simulink model "SMC_STA_HW_2_r2024b_test_2024"  (R2024b)
settings: Solver=FixedStepDiscrete  StartTime=0.0  StopTime=inf  FixedStep=0.002  RelTol=1e-3  EnableMultiTasking=on
PostLoadFcn:
  | qc_set_target_type(getConfigSet(bdroot, 'QUARC Default Target Configuration'));
undefined symbols (not defined in the file): HIL
libraries: quarc_library x4
settings Model: SimulationMode=external  ExtModeTrigDuration=5000  Creator=pmartin  LastModifiedBy=U448565
settings SolverCC: AlgebraicLoopSolver=TrustRegion  PositivePriorityOrder=on
settings DataIOCC: LimitDataPoints=on  SaveFormat=Array  SignalLoggingSaveFormat=ModelDataLogs  ReturnWorkspaceOutputs=off
settings OptimizationCC: ExpressionDepthLimit=2147483647  InitFltsAndDblsToZero=on
settings DebuggingCC: SaveWithParameterizedLinksMsg=none  UnderspecifiedInitializationDetection=Classic  MergeDetectMultiDrivingBlocksExec=none  SolverPrmCheckMsg=warning  MultiTaskDSMMsg=warning  MultiTaskCondExecSysMsg=none  FcnCallInpInsideContextMsg=warning  UnconnectedInputMsg=warning  UnconnectedOutputMsg=warning  UnconnectedLineMsg=warning  StateNameClashWarn=warning  SFUnexpectedBacktrackingDiag=warning  SFNoUnconditionalDefaultTransitionDiag=warning  SFExecutionAtInitializationDiag=none  ArithmeticOperatorsInVariantConditions=warning
settings ModelReferenceCC: PropagateSignalLabelsOutOfModel=off
settings SFSimCC: SimUseLocalCustomCode=off  CustomCodeUndefinedFunction=UseInterfaceOnly
settings RTWCC: Description=QUARC Win64 Target Using Toolchain  SystemTargetFile=quarc_win64.tlc  TemplateMakefile=quarc_default_tmf  RTWUseLocalCustomCode=off  Toolchain=QUARC win64 | nmake (64-bit Windows)  BuildConfiguration=Faster Runs  GPUComputeCapability=3.5
settings CodeAppCC: StateflowObjectComments=on
settings STFCustomTargetCC: ConcurrentExecutionCompliant=on  GRTInterface=on  UseToolchainInfoCompliant=on  SystemTargetFile=quarc_win64.tlc
settings GRTTargetCC: TargetLangStandard=C89/C90 (ANSI)  ParMdlRefBuildCompliant=off  CompOptLevelCompliant=off  CombineOutputUpdateFcns=off  MatFileLogging=off  CPPClassGenCompliant=off  GRTInterface=on  ExtMode=on  ExtModeMexFile=quarc_comm
settings ConfigComp: CovMetricSettings=dw  CovSaveCumulativeToWorkspaceVar=on  CovSaveSingleToWorkspaceVar=on  CovExternalEMLEnable=off  CovBoundaryAbsTol=1.0e-5

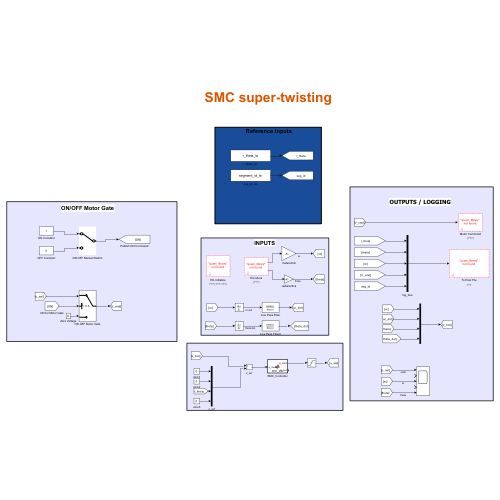
[thumbnail: Simulink's stored preview of the top-level diagram]
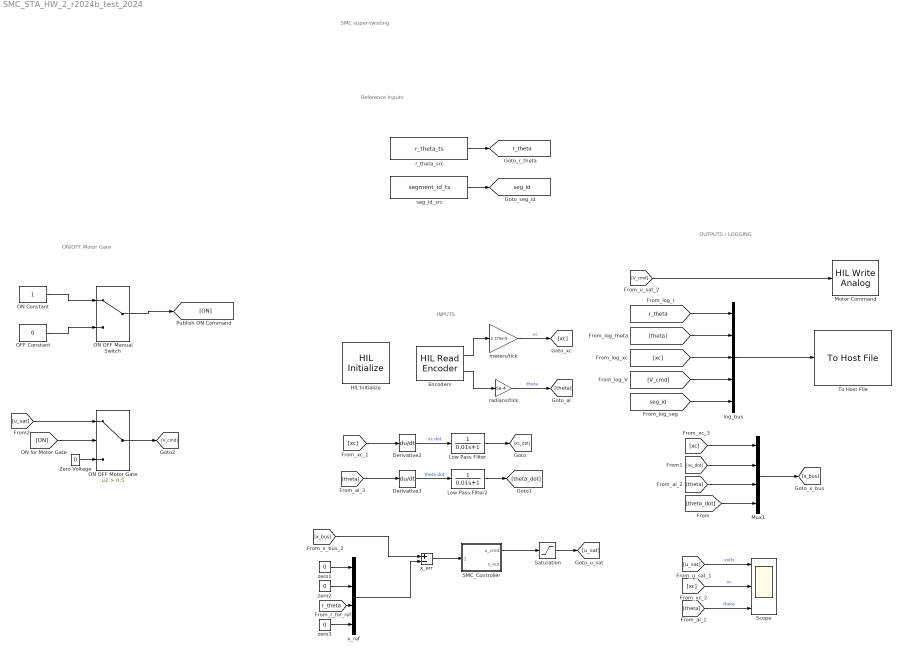
== system SMC_STA_HW_2_r2024b_test_2024 ==
  note: OUTPUTS / LOGGING
  note: INPUTS
  note: SMC super-twisting
  note: Reference Inputs
  note: ON/OFF Motor Gate
  Derivative2 : Derivative
  Derivative3 : Derivative
  Encoders : quarc_library/Data Acquisition/Generic/Immediate I//O/HIL Read Encoder  object_name=HIL-1  channels=[0:1]  sample_time=qc_get_step_size  active=on  vector_output=off  data_type_mode=Inherit via back propagation  data_type=double
  HIL Initialize : quarc_library/Data Acquisition/Generic/Configuration/HIL Initialize  object_name=HIL-1  board_type=q2_usb  board_number=0  board_options=d0=digital;d1=digital;led=auto;update_rate=normal  exclusive=off  active=off  hardware_clocks=[0:2]  clock_modes=[]  initial_clock_frequencies=[]  set_clock_params_at_start=off  set_clock_params_at_switch_in=off  set_clock_frequencies_at_start=off  set_clock_frequencies_at_switch_in=off  analog_input_channels=[0:1]  analog_input_configurations=[]  analog_input_maximums=10  analog_input_minimums=-10  set_analog_input_params_at_start=on  set_analog_input_params_at_switch_in=off  analog_output_channels=[0:1]  analog_output_maximums=10  analog_output_minimums=-10  initial_analog_outputs=[0]  final_analog_outputs=[0]  watchdog_analog_outputs=0  set_analog_output_params_at_start=on  set_analog_output_params_at_switch_in=off  set_analog_outputs_at_start=on  set_analog_outputs_at_switch_in=off  set_analog_outputs_at_terminate=on  set_analog_outputs_at_switch_out=off  set_analog_outputs_on_watchdog=off  digital_input_channels=[]  digital_output_channels=[0:7]  digital_output_configuration=[]  initial_digital_outputs=[0]  final_digital_outputs=[0]  watchdog_digital_outputs=[0]  set_digital_output_params_at_start=off  set_digital_output_params_at_switch_in=off  set_digital_outputs_at_start=on  set_digital_outputs_at_switch_in=off  set_digital_outputs_at_terminate=on  set_digital_outputs_at_switch_out=off  set_digital_outputs_on_watchdog=off  encoder_channels=[0:1]  quadrature=[4]  encoder_filter_frequency=[]  initial_encoder_counts=[0]  set_encoder_params_at_start=on  set_encoder_params_at_switch_in=off  set_encoder_counts_at_start=on  set_encoder_counts_at_switch_in=off  pwm_channels=[]  pwm_modes=[0]  pwm_frequency=1/0.020  pwm_configuration=[]  pwm_alignment=[]  pwm_polarity=[]  pwm_leading_deadband=[]  pwm_trailing_deadband=[]  initial_pwm_outputs=[0]  final_pwm_outputs=[0]  watchdog_pwm_outputs=[0]  set_pwm_params_at_start=on  set_pwm_params_at_switch_in=off  set_pwm_outputs_at_start=on  set_pwm_outputs_at_switch_in=off  set_pwm_outputs_at_terminate=on  set_pwm_outputs_at_switch_out=off  set_pwm_outputs_on_watchdog=off  other_output_channels=[]  initial_other_outputs=[]  final_other_outputs=[]  watchdog_other_outputs=[]  set_other_outputs_at_start=off  set_other_outputs_at_switch_in=off  set_other_outputs_at_terminate=off  set_other_outputs_at_switch_out=off  set_other_outputs_on_watchdog=off
  Low Pass Filter : TransferFcn  Denominator=[0.01 1]
  Low Pass Filter2 : TransferFcn  Denominator=[0.01 1]
  Motor Command : quarc_library/Data Acquisition/Generic/Immediate I//O/HIL Write Analog  object_name=HIL-1  channels=0  sample_time=-1  active=off  vector_input=off
  Mux1 : Mux
  OFF Constant : Constant  Value=0
  ON Constant : Constant
  ON OFF Manual Switch : ManualSwitch
  ON OFF Motor Gate : Switch  Criteria=u2 > Threshold  Threshold=0.5  SaturateOnIntegerOverflow=off  InputSameDT=off
  SMC_Controller : MATLAB Function  Description=Super-Twisting SMC (second-order sliding mode, after STA). Continuous voltage command via integrator state v. u = -K_eq*x + (-k1*sqrt(|s|)*sat(s/phi) + v)/(S*B), v_dot = -k2*sat(s/phi).  TreatAsAtomicUnit=on
  Saturation : Saturate  UpperLimit=6  LowerLimit=-6
  Scope : Scope  NumInputPorts=5
  To Host File : quarc_library/Sinks/To Host/To Host File  source=Specify via dialog (do not evaluate)  file_name=data_%{date}_%{time}.mat  variable_name=data  decimation=1  sample_time=-1  file_format=MAT-file v.4  options=No header or footer  append=off  final_file_name=data_05-May-2026_17-28-00.mat  encoding=Default  bitrate=0
  Zero Voltage : Constant  Value=0
  log_bus : Mux  Inputs=5
  meters/tick : Gain  Gain=2.275e-5
  r_theta_src : FromWorkspace  VariableName=r_theta_ts  OutputAfterFinalValue=Holding final value
  radians/tick : Gain  Gain=5e-4
  seg_id_src : FromWorkspace  VariableName=segment_id_ts  Interpolate=off  OutputAfterFinalValue=Holding final value
  x_err : Sum  Inputs=+-
  x_ref : Mux
  zero1 : Constant  Value=0
  zero2 : Constant  Value=0
  zero3 : Constant  Value=0
  tag scope: r_theta=global, seg_id=global
  wires:
  meters/tick/1 -> [xc]  "xc"
  Encoders/1 -> meters/tick/1
  Encoders/2 -> radians/tick/1
  [V_cmd] -> Motor Command/1
  [xc] -> Derivative2/1
  [theta] -> Derivative3/1
  radians/tick/1 -> [theta]  "theta"
  SMC_Controller/1(u_cmd) -> Saturation/1
  Derivative2/1 -> Low Pass Filter/1  "xc dot"
  Derivative3/1 -> Low Pass Filter2/1  "theta dot"
  [xc] -> Mux1/1
  Saturation/1 -> [u_sat]
  [theta] -> Mux1/3
  [u_sat] -> Scope/1  "volts"
  Mux1/1 -> [x_bus]
  Low Pass Filter/1 -> [xc_dot]
  Low Pass Filter2/1 -> [theta_dot]
  [theta_dot] -> Mux1/4
  [xc_dot] -> Mux1/2
  [xc] -> Scope/3  "xc"
  [theta] -> Scope/5  "theta"
  r_theta_src/1 -> [r_theta]
  seg_id_src/1 -> [seg_id]
  zero1/1 -> x_ref/1
  zero2/1 -> x_ref/2
  [r_theta] -> x_ref/3
  zero3/1 -> x_ref/4
  [x_bus] -> x_err/1
  x_ref/1 -> x_err/2
  x_err/1 -> SMC_Controller/1(x_meas)
  [r_theta] -> log_bus/1
  [theta] -> log_bus/2
  [xc] -> log_bus/3
  [V_cmd] -> log_bus/4
  [seg_id] -> log_bus/5
  log_bus/1 -> To Host File/1
  ON OFF Manual Switch/1 -> [ON]
  ON OFF Motor Gate/1 -> [V_cmd]
  ON Constant/1 -> ON OFF Manual Switch/1
  Zero Voltage/1 -> ON OFF Motor Gate/3
  [u_sat] -> ON OFF Motor Gate/1
  OFF Constant/1 -> ON OFF Manual Switch/2
  [ON] -> ON OFF Motor Gate/2

== matlab function SMC_STA_HW_2_r2024b_test_2024/SMC_Controller ==
  settings: updateMethod=DISCRETE  sampleTime=0.002
  data: x_meas input; u_cmd output; s_out output
function [u_cmd, s_out] = smc_sta(x_meas)
%#codegen
% Super-Twisting SMC (after STA): continuous-output reaching law.
% Persistent integrator state v advances each sample.  Boundary-layer
% sat(s/phi) replaces sign(s) to handle encoder quantization.
%
%   u     = -K_eq*x + ( -k1*sqrt(max(|s|,phi))*sat(s/phi) + v ) / (S*B)
%   v_dot = -k2 * sat(s/phi)        (forward-Euler integration)

    persistent v
    if isempty(v), v = 0; end

    Ts     = 0.002;
    S      = [17.93844926, 2.150758485, -29.94418177, -9.949392121];
    K_eq   = [30.77536055, -6.546877011, -24.23551815, -10.39621569];
    k1     = 6.363961031;
    k2     = 19.8;
    phi    = 0.03845047651;

    s   = S * x_meas(:);
    sig = max(min(s/max(phi, eps), 1), -1);

    % reaching law
    SB    = 2.880296318;          % precomputed S*B
    u_sw  = (-k1 * sqrt(max(abs(s), phi)) * sig + v) / SB;

    % integrator update (forward Euler)
    v_dot = -k2 * sig;
    v     = v + Ts * v_dot;

    % combine + saturate
    u_cmd     = -K_eq * x_meas(:) + u_sw;
    s_out = s;
end
